simulink model "Universal_Convert_1"  (R2025a)
settings: Solver=VariableStepAuto  StartTime=0.0  StopTime=10.0  RelTol=1e-3
settings Model: LastModifiedBy=Johan

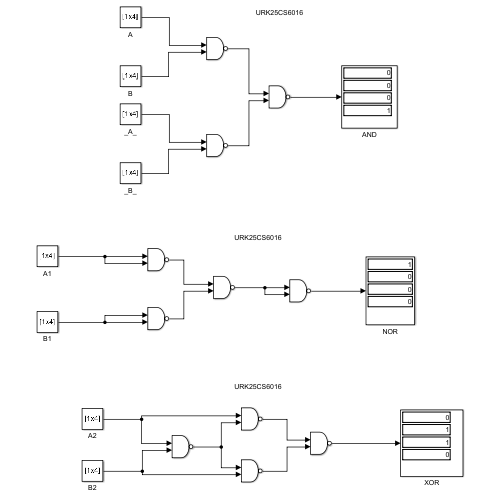
[thumbnail: Simulink's stored preview of the top-level diagram]
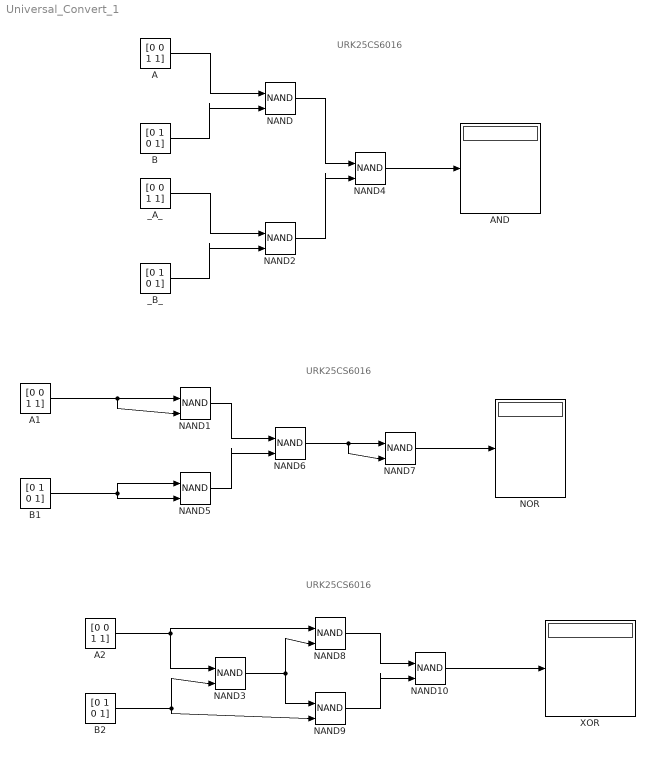
== system Universal_Convert_1 ==
  note: URK25CS6016
  note: URK25CS6016
  note: URK25CS6016
  A : Constant  Value=[0 0 1 1]
  A1 : Constant  Value=[0 0 1 1]
  A2 : Constant  Value=[0 0 1 1]
  AND : Display
  B : Constant  Value=[0 1 0 1]
  B1 : Constant  Value=[0 1 0 1]
  B2 : Constant  Value=[0 1 0 1]
  NAND{,1..10} (11 alike) : Logic  Operator=NAND  IconShape=distinctive  AllPortsSameDT=off  OutDataTypeStr=boolean
  NOR : Display
  XOR : Display
  _A_ : Constant  Value=[0 0 1 1]
  _B_ : Constant  Value=[0 1 0 1]
  wires:
  A/1 -> NAND/1
  B/1 -> NAND/2
  A1/1 -> NAND1/2, NAND1/1
  B2/1 -> NAND3/2, NAND9/2
  A2/1 -> NAND8/1, NAND3/1
  _A_/1 -> NAND2/1
  _B_/1 -> NAND2/2
  NAND/1 -> NAND4/1
  NAND2/1 -> NAND4/2
  NAND4/1 -> AND/1
  B1/1 -> NAND5/1, NAND5/2
  NAND1/1 -> NAND6/1
  NAND5/1 -> NAND6/2
  NAND6/1 -> NAND7/2, NAND7/1
  NAND7/1 -> NOR/1
  NAND3/1 -> NAND8/2, NAND9/1
  NAND8/1 -> NAND10/1
  NAND9/1 -> NAND10/2
  NAND10/1 -> XOR/1
